simulink model "uavsim_trim"  (R2022a)
settings: Solver=VariableStepAuto  StartTime=0.0  StopTime=10.0  RelTol=1e-3
undefined symbols (not defined in the file or in its folder): forces_moments, UAV
settings Model: Creator=20066227d  LastModifiedBy=20066227d
settings DebuggingCC: InitInArrayFormatMsg=none

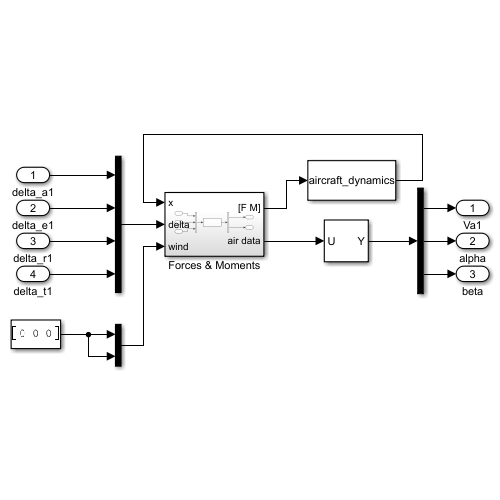
[thumbnail: Simulink's stored preview of the top-level diagram]
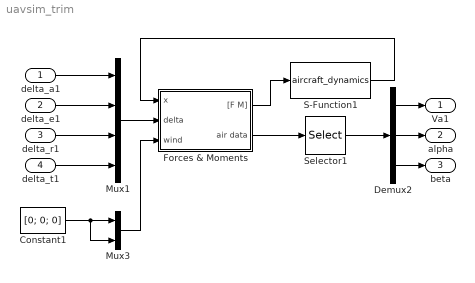
== system uavsim_trim ==
  delta_a1 : Inport
  delta_e1 : Inport  Port=2
  delta_r1 : Inport  Port=3
  delta_t1 : Inport  Port=4
  Constant1 : Constant  Value=[0; 0; 0]
  Demux2 : Demux  Outputs=3
  Forces & Moments : Subsystem
  Mux1 : Mux
  Mux3 : Mux  Inputs=2
  S-Function1 : S-Function  FunctionName=aircraft_dynamics  Parameters=UAV  SFunctionDeploymentMode=off  EnableBusSupport=off
  Selector1 : Selector  InputPortWidth=6  IndexOptions=Index vector (dialog)  Indices=[1 2 3]  OutputSizes=1
  Va1 : Outport
  alpha : Outport  Port=2
  beta : Outport  Port=3
  wires:
  S-Function1/1 -> Forces & Moments/1(x)
  Mux1/1 -> Forces & Moments/2(delta)
  delta_e1/1 -> Mux1/2
  delta_a1/1 -> Mux1/1
  delta_t1/1 -> Mux1/4
  Selector1/1 -> Demux2/1
  delta_r1/1 -> Mux1/3
  Constant1/1 -> Mux3/1, Mux3/2
  Demux2/2 -> alpha/1
  Demux2/1 -> Va1/1
  Mux3/1 -> Forces & Moments/3(wind)
  Forces & Moments/1("[F M]") -> S-Function1/1
  Demux2/3 -> beta/1
  Forces & Moments/2(air data) -> Selector1/1

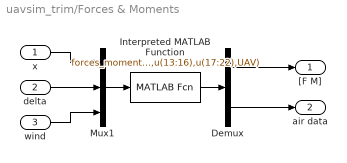
== system uavsim_trim/Forces & Moments ==
  x : Inport
  delta : Inport  Port=2
  wind : Inport  Port=3
  Demux : Demux  Outputs=[6;6]
  Interpreted MATLAB Function : MATLABFcn  MATLABFcn=forces_moments(u(1:12),u(13:16),u(17:22),UAV)  OutputDimensions=12
  Mux1 : Mux  Inputs=3
  "[F M]" : Outport
  air data : Outport  Port=2
  wires:
  Interpreted MATLAB Function/1 -> Demux/1
  Demux/2 -> air data/1
  x/1 -> Mux1/1
  Mux1/1 -> Interpreted MATLAB Function/1
  Demux/1 -> "[F M]"/1
  delta/1 -> Mux1/2
  wind/1 -> Mux1/3
